simulink model "controllo_cascata_2019"  (R2019b)
settings: Solver=VariableStepAuto  StartTime=0.0  StopTime=5  RelTol=1e-3
values from neighbouring files (symbols this model uses):
  den = den{1}    [Km_con_filtri.m]    (also in fft_signal_analysis.m)
  Gden = Gden{1}    [controllore_mag_lin.m]
  Gnum = Gnum{1}    [controllore_mag_lin.m]
  ki = 2117.9265    [controller_el.m]    (also in controller_el_windup.m; controllore_el2.m = 104; controllore_mag_lin.m; validation_controller_freq.m = 2118)
  kp = 46.0161    [controller_el.m]    (also in controller_el_windup.m; controllore_el2.m = 0.15; controllore_mag_lin.m; validation_controller_freq.m = 46)
  Lc = 0.3935    [Model_Parameter.m]    (also in Model_Parameter_version2.m = 0.3708; Stima_dei_parametri_Rc_Lc.m = mean(Lc_vect))
  num = num{1}    [Km_con_filtri.m]    (also in fft_signal_analysis.m)
  Rtot = 9.089    [Model_Parameter.m]    (also in Model_Parameter_version2.m = 9.7585)
undefined symbols (not defined in the file or in its folder): den_ext, den_unico, dist, Gdclose, Gnclose, num_ext, num_unico, u0, x10, x1_eq
libraries: simulink x5
settings Model: Creator=lollo  LastModifiedBy=lollo
settings DebuggingCC: UnconnectedInputMsg=none  UnconnectedOutputMsg=none  UnconnectedLineMsg=none
settings ModelReferenceCC: EnableRefExpFcnMdlSchedulingChecks=off
settings RTWCC: Description=Generic Real-Time Target

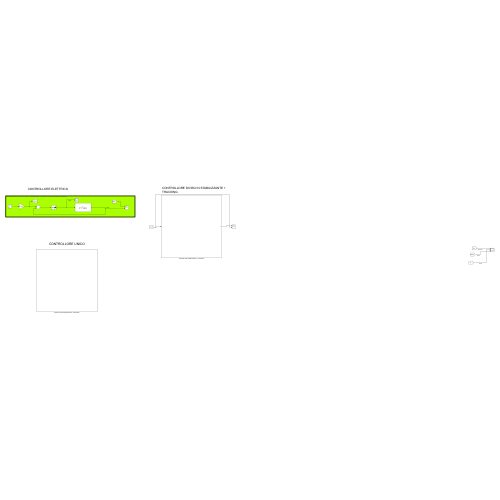
[thumbnail: Simulink's stored preview of the top-level diagram]
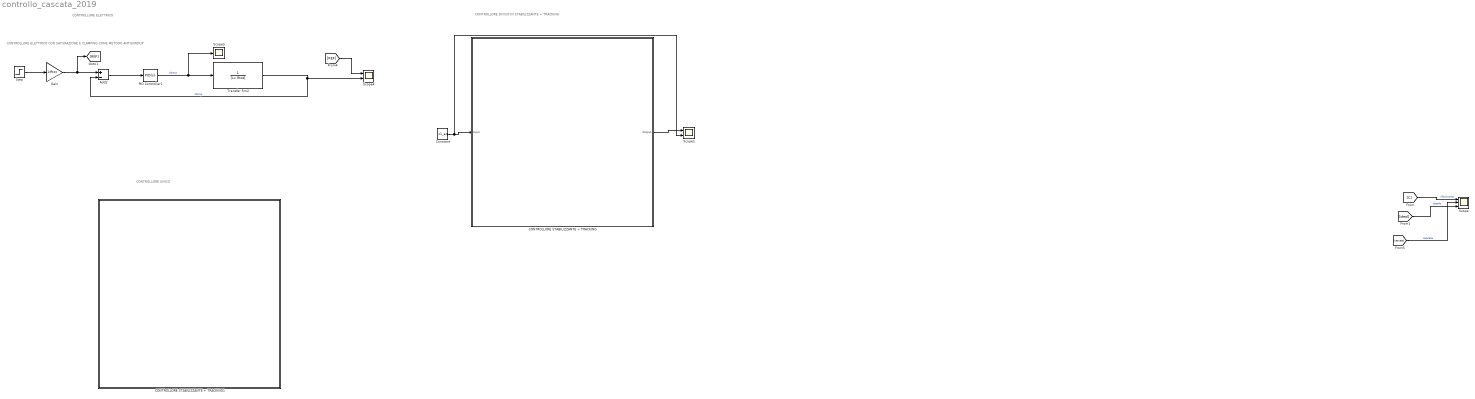
== system controllo_cascata_2019 ==
  note: CONTROLLORE UNICO
  note: CONTROLLORE ELETTRICO
  note: CONTROLLORE DIVISO IN STABILIZZANTE + TRACKING
  note: CONTROLLORE ELETTRICO CON SATURAZIONE E CLAMPING COME METODO ANTIWINDUP
  Add2 : Sum  Inputs=+-
  CONTROLLORE STABILIZZANTE + TRACKING : Subsystem
  CONTROLLORE STABILIZZANTE + TRACKING1 : Subsystem
  Constant : Constant  Value=x1_eq
  Gain : Gain  Gain=1/Rtot
  PID Controller1 : simulink/Continuous/PID Controller  Controller=PID  Form=Parallel  TimeDomain=Continuous-time  SampleTime=-1  IntegratorMethod=Forward Euler  FilterMethod=Forward Euler  ControllerParametersSource=internal  P=kp  I=ki  D=0  N=100  UseFilter=on  TunerSelectOption=Transfer Function Based (PID Tuner App)  InitialConditionSource=internal  InitialConditionForIntegrator=0  InitialConditionForFilter=0  DifferentiatorICPrevScaledInput=0  ExternalReset=none  TrackingMode=off  Kt=1  LimitOutput=on  UpperSaturationLimit=23  LowerSaturationLimit=-23  LinearizeAsGain=on  AntiWindupMode=clamping  Kb=1  POutMin=[]  POutMax=[]  IOutMin=[]  IOutMax=[]  DOutMin=[]  DOutMax=[]  NOutMin=[]  NOutMax=[]  SumOutMin=[]  SumOutMax=[]  SaturationOutMin=[]  SaturationOutMax=[]  PParamMin=[]  PParamMax=[]  IParamMin=[]  IParamMax=[]  DParamMin=[]  DParamMax=[]  NParamMin=[]  NParamMax=[]  KbParamMin=[]  KbParamMax=[]  KtParamMin=[]  KtParamMax=[]  KbOutMin=[]  KbOutMax=[]  KtOutMin=[]  KtOutMax=[]  IntegratorOutMin=[]  IntegratorOutMax=[]  FilterOutMin=[]  FilterOutMax=[]  SumI1OutMin=[]  SumI1OutMax=[]  SumI2OutMin=[]  SumI2OutMax=[]  SumI3OutMin=[]  SumI3OutMax=[]  SumI4OutMin=[]  SumI4OutMax=[]  SumDOutMin=[]  SumDOutMax=[]  DifferentiatorOutMin=[]  DifferentiatorOutMax=[]  FilterDiffOutCoefMin=[]  FilterDiffOutCoefMax=[]  ReciprocalOutMin=[]  ReciprocalOutMax=[]  SumDenOutMin=[]  SumDenOutMax=[]  SumNumOutMin=[]  SumNumOutMax=[]  DivideOutMin=[]  DivideOutMax=[]  IntegratorContinuousStateAttributes=''  IntegratorStateMustResolveToSignalObject=off  IntegratorRTWStateStorageClass=Auto  FilterContinuousStateAttributes=''  FilterStateMustResolveToSignalObject=off  FilterRTWStateStorageClass=Auto  ParallelPVariant=InternalParameters  IdealPVariant=Disabled  IVariant=InternalParameters  DVariant=InternalParameters  IntegratorVariant=Continuous  SatVariant=Enabled  AWVariant=ContClampingParallel  PCopyVariant=Disabled  TRVariant=Disabled  FdbkBlocksVariant=Forward  IdealPFdbkVariant=Disabled  SatFdbkVariant=Disabled  DerivativeFilterVariant=ContFilter  NVariant=InternalParameters  NCopyVariant=Disabled  FilterICVariant=InternalICsFilter  IntegratorICVariant=InternalICs  ExternalResetVariant=Disabled  TRSumVariant=Passthrough  SumFdbkVariant=Disabled  SumVariant=Sum_PID
  Scope : Scope  NumInputPorts=3
  Scope1 : Scope  NumInputPorts=2
  Scope4 : Scope  NumInputPorts=2
  Scope5 : Scope
  Step : Step  Time=0  After=10  SampleTime=0
  Transfer Fcn2 : TransferFcn  Denominator=[Lc Rtot]
  wires:
  Add2/1 -> PID Controller1/1
  PID Controller1/1 -> Scope5/1, Transfer Fcn2/1  "clamp"
  Transfer Fcn2/1 -> Scope4/2, Add2/2  "clamp"
  Step/1 -> Gain/1
  [REF] -> Scope4/1
  [C] -> Scope/1  "riferimenti"
  [ideal] -> Scope/3  "ideale"
  [cascata] -> Scope/2  "cascata"
  Gain/1 -> [REF], Add2/1
  Constant/1 -> Scope1/2, CONTROLLORE STABILIZZANTE + TRACKING/1(Input)
  CONTROLLORE STABILIZZANTE + TRACKING/1(Output) -> Scope1/1

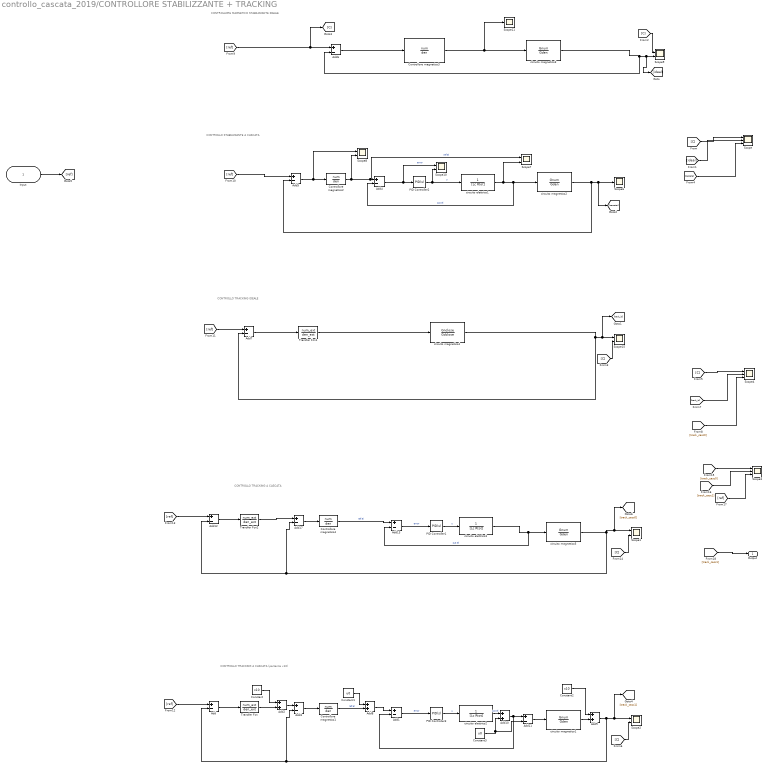
== system controllo_cascata_2019/CONTROLLORE STABILIZZANTE + TRACKING ==
  note: CONTROLLO STABILIZZANTE A CASCATA
  note: CONTROLLORE MAGNETICO STABILIZZANTE IDEALE
  note: CONTROLLO TRACKING A CASCATA (partenza x10)
  note: CONTROLLO TRACKING IDEALE
  note: CONTROLLO TRACKING A CASCATA
  Input : Inport
  Add{,1,3..7,11..13,17} (11 alike) : Sum  Inputs=+-
  Add{2,8..10} (4 alike) : Sum
  Constant : Constant  Value=x10
  Constant1 : Constant  Value=u0
  Constant2 : Constant  Value=x10
  Constant3 : Constant  Value=u0
  Controllore magnetico{1..4} (4 alike) : TransferFcn  Numerator=num  Denominator=den
  PID Controller1 : simulink/Continuous/PID Controller  Controller=PID  Form=Parallel  TimeDomain=Continuous-time  SampleTime=-1  IntegratorMethod=Forward Euler  FilterMethod=Forward Euler  ControllerParametersSource=internal  P=kp  I=ki  D=0  N=100  UseFilter=on  TunerSelectOption=Transfer Function Based (PID Tuner App)  InitialConditionSource=internal  InitialConditionForIntegrator=0  InitialConditionForFilter=0  DifferentiatorICPrevScaledInput=0  ExternalReset=none  TrackingMode=off  Kt=1  LimitOutput=on  UpperSaturationLimit=23  LowerSaturationLimit=-23  LinearizeAsGain=on  AntiWindupMode=clamping  Kb=1  POutMin=[]  POutMax=[]  IOutMin=[]  IOutMax=[]  DOutMin=[]  DOutMax=[]  NOutMin=[]  NOutMax=[]  SumOutMin=[]  SumOutMax=[]  SaturationOutMin=[]  SaturationOutMax=[]  PParamMin=[]  PParamMax=[]  IParamMin=[]  IParamMax=[]  DParamMin=[]  DParamMax=[]  NParamMin=[]  NParamMax=[]  KbParamMin=[]  KbParamMax=[]  KtParamMin=[]  KtParamMax=[]  KbOutMin=[]  KbOutMax=[]  KtOutMin=[]  KtOutMax=[]  IntegratorOutMin=[]  IntegratorOutMax=[]  FilterOutMin=[]  FilterOutMax=[]  SumI1OutMin=[]  SumI1OutMax=[]  SumI2OutMin=[]  SumI2OutMax=[]  SumI3OutMin=[]  SumI3OutMax=[]  SumI4OutMin=[]  SumI4OutMax=[]  SumDOutMin=[]  SumDOutMax=[]  DifferentiatorOutMin=[]  DifferentiatorOutMax=[]  FilterDiffOutCoefMin=[]  FilterDiffOutCoefMax=[]  ReciprocalOutMin=[]  ReciprocalOutMax=[]  SumDenOutMin=[]  SumDenOutMax=[]  SumNumOutMin=[]  SumNumOutMax=[]  DivideOutMin=[]  DivideOutMax=[]  IntegratorContinuousStateAttributes=''  IntegratorStateMustResolveToSignalObject=off  IntegratorRTWStateStorageClass=Auto  FilterContinuousStateAttributes=''  FilterStateMustResolveToSignalObject=off  FilterRTWStateStorageClass=Auto  ParallelPVariant=InternalParameters  IdealPVariant=Disabled  IVariant=InternalParameters  DVariant=InternalParameters  IntegratorVariant=Continuous  SatVariant=Enabled  AWVariant=ContClampingParallel  PCopyVariant=Disabled  TRVariant=Disabled  FdbkBlocksVariant=Forward  IdealPFdbkVariant=Disabled  SatFdbkVariant=Disabled  DerivativeFilterVariant=ContFilter  NVariant=InternalParameters  NCopyVariant=Disabled  FilterICVariant=InternalICsFilter  IntegratorICVariant=InternalICs  ExternalResetVariant=Disabled  TRSumVariant=Passthrough  SumFdbkVariant=Disabled  SumVariant=Sum_PID
  PID Controller2 : simulink/Continuous/PID Controller  Controller=PID  Form=Parallel  TimeDomain=Continuous-time  SampleTime=-1  IntegratorMethod=Forward Euler  FilterMethod=Forward Euler  ControllerParametersSource=internal  P=kp  I=ki  D=0  N=100  UseFilter=on  TunerSelectOption=Transfer Function Based (PID Tuner App)  InitialConditionSource=internal  InitialConditionForIntegrator=0  InitialConditionForFilter=0  DifferentiatorICPrevScaledInput=0  ExternalReset=none  TrackingMode=off  Kt=1  LimitOutput=on  UpperSaturationLimit=23  LowerSaturationLimit=-23  LinearizeAsGain=on  AntiWindupMode=clamping  Kb=1  POutMin=[]  POutMax=[]  IOutMin=[]  IOutMax=[]  DOutMin=[]  DOutMax=[]  NOutMin=[]  NOutMax=[]  SumOutMin=[]  SumOutMax=[]  SaturationOutMin=[]  SaturationOutMax=[]  PParamMin=[]  PParamMax=[]  IParamMin=[]  IParamMax=[]  DParamMin=[]  DParamMax=[]  NParamMin=[]  NParamMax=[]  KbParamMin=[]  KbParamMax=[]  KtParamMin=[]  KtParamMax=[]  KbOutMin=[]  KbOutMax=[]  KtOutMin=[]  KtOutMax=[]  IntegratorOutMin=[]  IntegratorOutMax=[]  FilterOutMin=[]  FilterOutMax=[]  SumI1OutMin=[]  SumI1OutMax=[]  SumI2OutMin=[]  SumI2OutMax=[]  SumI3OutMin=[]  SumI3OutMax=[]  SumI4OutMin=[]  SumI4OutMax=[]  SumDOutMin=[]  SumDOutMax=[]  DifferentiatorOutMin=[]  DifferentiatorOutMax=[]  FilterDiffOutCoefMin=[]  FilterDiffOutCoefMax=[]  ReciprocalOutMin=[]  ReciprocalOutMax=[]  SumDenOutMin=[]  SumDenOutMax=[]  SumNumOutMin=[]  SumNumOutMax=[]  DivideOutMin=[]  DivideOutMax=[]  IntegratorContinuousStateAttributes=''  IntegratorStateMustResolveToSignalObject=off  IntegratorRTWStateStorageClass=Auto  FilterContinuousStateAttributes=''  FilterStateMustResolveToSignalObject=off  FilterRTWStateStorageClass=Auto  ParallelPVariant=InternalParameters  IdealPVariant=Disabled  IVariant=InternalParameters  DVariant=InternalParameters  IntegratorVariant=Continuous  SatVariant=Enabled  AWVariant=ContClampingParallel  PCopyVariant=Disabled  TRVariant=Disabled  FdbkBlocksVariant=Forward  IdealPFdbkVariant=Disabled  SatFdbkVariant=Disabled  DerivativeFilterVariant=ContFilter  NVariant=InternalParameters  NCopyVariant=Disabled  FilterICVariant=InternalICsFilter  IntegratorICVariant=InternalICs  ExternalResetVariant=Disabled  TRSumVariant=Passthrough  SumFdbkVariant=Disabled  SumVariant=Sum_PID
  PID Controller3 : simulink/Continuous/PID Controller  Controller=PID  Form=Parallel  TimeDomain=Continuous-time  SampleTime=-1  IntegratorMethod=Forward Euler  FilterMethod=Forward Euler  ControllerParametersSource=internal  P=kp  I=ki  D=0  N=100  UseFilter=on  TunerSelectOption=Transfer Function Based (PID Tuner App)  InitialConditionSource=internal  InitialConditionForIntegrator=0  InitialConditionForFilter=0  DifferentiatorICPrevScaledInput=0  ExternalReset=none  TrackingMode=off  Kt=1  LimitOutput=on  UpperSaturationLimit=23  LowerSaturationLimit=-23  LinearizeAsGain=on  AntiWindupMode=clamping  Kb=1  POutMin=[]  POutMax=[]  IOutMin=[]  IOutMax=[]  DOutMin=[]  DOutMax=[]  NOutMin=[]  NOutMax=[]  SumOutMin=[]  SumOutMax=[]  SaturationOutMin=[]  SaturationOutMax=[]  PParamMin=[]  PParamMax=[]  IParamMin=[]  IParamMax=[]  DParamMin=[]  DParamMax=[]  NParamMin=[]  NParamMax=[]  KbParamMin=[]  KbParamMax=[]  KtParamMin=[]  KtParamMax=[]  KbOutMin=[]  KbOutMax=[]  KtOutMin=[]  KtOutMax=[]  IntegratorOutMin=[]  IntegratorOutMax=[]  FilterOutMin=[]  FilterOutMax=[]  SumI1OutMin=[]  SumI1OutMax=[]  SumI2OutMin=[]  SumI2OutMax=[]  SumI3OutMin=[]  SumI3OutMax=[]  SumI4OutMin=[]  SumI4OutMax=[]  SumDOutMin=[]  SumDOutMax=[]  DifferentiatorOutMin=[]  DifferentiatorOutMax=[]  FilterDiffOutCoefMin=[]  FilterDiffOutCoefMax=[]  ReciprocalOutMin=[]  ReciprocalOutMax=[]  SumDenOutMin=[]  SumDenOutMax=[]  SumNumOutMin=[]  SumNumOutMax=[]  DivideOutMin=[]  DivideOutMax=[]  IntegratorContinuousStateAttributes=''  IntegratorStateMustResolveToSignalObject=off  IntegratorRTWStateStorageClass=Auto  FilterContinuousStateAttributes=''  FilterStateMustResolveToSignalObject=off  FilterRTWStateStorageClass=Auto  ParallelPVariant=InternalParameters  IdealPVariant=Disabled  IVariant=InternalParameters  DVariant=InternalParameters  IntegratorVariant=Continuous  SatVariant=Enabled  AWVariant=ContClampingParallel  PCopyVariant=Disabled  TRVariant=Disabled  FdbkBlocksVariant=Forward  IdealPFdbkVariant=Disabled  SatFdbkVariant=Disabled  DerivativeFilterVariant=ContFilter  NVariant=InternalParameters  NCopyVariant=Disabled  FilterICVariant=InternalICsFilter  IntegratorICVariant=InternalICs  ExternalResetVariant=Disabled  TRSumVariant=Passthrough  SumFdbkVariant=Disabled  SumVariant=Sum_PID
  Scope : Scope  NumInputPorts=3
  Scope{1..2,7..10,15} (7 alike) : Scope  NumInputPorts=2
  Scope11 : Scope
  Scope3 : Scope  NumInputPorts=3
  Scope4 : Scope  NumInputPorts=3
  Scope6 : Scope
  Transfer Fcn : TransferFcn  Numerator=num_ext  Denominator=den_ext
  Transfer Fcn1 : TransferFcn  Numerator=num_ext  Denominator=den_ext
  Transfer Fcn2 : TransferFcn  Numerator=num_ext  Denominator=den_ext
  circuito elettrico1 : TransferFcn  Denominator=[Lc Rtot]
  circuito elettrico2 : TransferFcn  Denominator=[Lc Rtot]
  circuito elettrico3 : TransferFcn  Denominator=[Lc Rtot]
  circuito magnetico{1..3,5} (4 alike) : TransferFcn  Numerator=Gnum  Denominator=Gden
  circuito magnetico4 : TransferFcn  Numerator=Gnclose  Denominator=Gdclose
  Output : Outport
  wires:
  circuito magnetico2/1 -> Add5/2, [cascata], Scope6/1
  circuito elettrico1/1 -> Scope7/2, Add4/2, circuito magnetico2/1  "out el"
  Add4/1 -> Scope10/1, PID Controller2/1  "error"
  Controllore magnetico2/1 -> Scope8/2, Scope7/1, Add4/1  "ref el"
  PID Controller3/1 -> circuito elettrico2/1  "u"
  [ref] -> Add/1
  Add5/1 -> Scope8/1, Controllore magnetico2/1
  Transfer Fcn1/1 -> circuito magnetico4/1
  Add3/1 -> Controllore magnetico1/1
  Add/1 -> Transfer Fcn/1
  [ref] -> Add5/1
  circuito magnetico4/1 -> Add7/2, [track_id], Scope15/1
  PID Controller2/1 -> Scope10/2, circuito elettrico1/1  "u"
  Add6/1 -> Controllore magnetico3/1
  [ref] -> [C], Add6/1
  circuito magnetico3/1 -> Add6/2, [ideal], Scope9/2
  Controllore magnetico3/1 -> Scope11/1, circuito magnetico3/1
  Add1/1 -> PID Controller3/1  "error"
  [C] -> Scope9/1
  [ref] -> Add7/1
  [C] -> Scope15/2
  Add7/1 -> Transfer Fcn1/1
  [C] -> Scope2/2
  [C] -> Scope/1
  [ideal] -> Scope/2
  [cascata] -> Scope/3
  [C] -> Scope4/1
  [track_id] -> Scope4/2
  [track_casc0] -> Scope4/3
  Input/1 -> [ref]
  Transfer Fcn/1 -> Add2/2
  Add2/1 -> Add3/1
  Constant/1 -> Add2/1
  Add8/1 -> Add1/1
  Controllore magnetico1/1 -> Add8/2  "ref el"
  Constant1/1 -> Add8/1
  Add9/1 -> [track_casc1], Scope2/1, Add3/2, Add/2
  circuito magnetico1/1 -> Add9/2
  Constant2/1 -> Add9/1
  Add11/1 -> circuito magnetico1/1
  circuito elettrico2/1 -> Add10/1  "out el"
  Add10/1 -> Add1/2, Add11/1
  Constant3/1 -> Add11/2, Add10/2
  [ref] -> Add12/1
  Controllore magnetico4/1 -> Add13/1  "ref el"
  circuito elettrico3/1 -> Add13/2, circuito magnetico5/1  "out el"
  circuito magnetico5/1 -> [track_casc0], Scope1/1, Add17/2, Add12/2
  Transfer Fcn2/1 -> Add17/1
  Add12/1 -> Transfer Fcn2/1
  [C] -> Scope1/2
  Add17/1 -> Controllore magnetico4/1
  PID Controller1/1 -> circuito elettrico3/1  "u"
  Add13/1 -> PID Controller1/1  "error"
  [track_casc0] -> Scope3/1
  [track_casc1] -> Scope3/2
  [ref] -> Scope3/3
  [track_casc1] -> Output/1

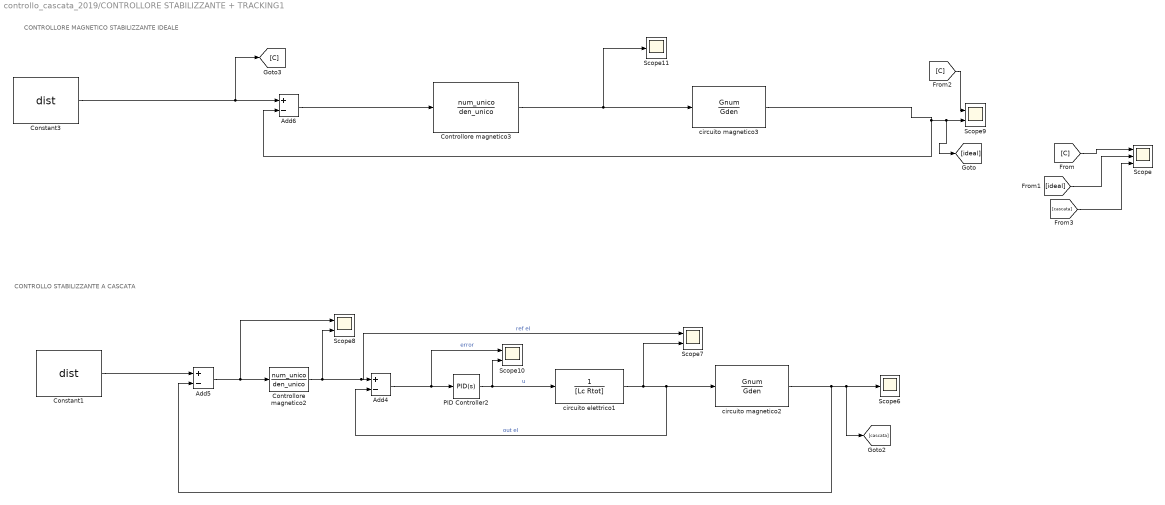
== system controllo_cascata_2019/CONTROLLORE STABILIZZANTE + TRACKING1 ==
  note: CONTROLLO STABILIZZANTE A CASCATA
  note: CONTROLLORE MAGNETICO STABILIZZANTE IDEALE
  Add4 : Sum  Inputs=+-
  Add5 : Sum  Inputs=+-
  Add6 : Sum  Inputs=+-
  Constant1 : Constant  Value=dist
  Constant3 : Constant  Value=dist
  Controllore magnetico2 : TransferFcn  Numerator=num_unico  Denominator=den_unico
  Controllore magnetico3 : TransferFcn  Numerator=num_unico  Denominator=den_unico
  PID Controller2 : simulink/Continuous/PID Controller  Controller=PID  Form=Parallel  TimeDomain=Continuous-time  SampleTime=-1  IntegratorMethod=Forward Euler  FilterMethod=Forward Euler  ControllerParametersSource=internal  P=kp  I=ki  D=0  N=100  UseFilter=on  TunerSelectOption=Transfer Function Based (PID Tuner App)  InitialConditionSource=internal  InitialConditionForIntegrator=0  InitialConditionForFilter=0  DifferentiatorICPrevScaledInput=0  ExternalReset=none  TrackingMode=off  Kt=1  LimitOutput=on  UpperSaturationLimit=23  LowerSaturationLimit=-23  LinearizeAsGain=on  AntiWindupMode=clamping  Kb=1  POutMin=[]  POutMax=[]  IOutMin=[]  IOutMax=[]  DOutMin=[]  DOutMax=[]  NOutMin=[]  NOutMax=[]  SumOutMin=[]  SumOutMax=[]  SaturationOutMin=[]  SaturationOutMax=[]  PParamMin=[]  PParamMax=[]  IParamMin=[]  IParamMax=[]  DParamMin=[]  DParamMax=[]  NParamMin=[]  NParamMax=[]  KbParamMin=[]  KbParamMax=[]  KtParamMin=[]  KtParamMax=[]  KbOutMin=[]  KbOutMax=[]  KtOutMin=[]  KtOutMax=[]  IntegratorOutMin=[]  IntegratorOutMax=[]  FilterOutMin=[]  FilterOutMax=[]  SumI1OutMin=[]  SumI1OutMax=[]  SumI2OutMin=[]  SumI2OutMax=[]  SumI3OutMin=[]  SumI3OutMax=[]  SumI4OutMin=[]  SumI4OutMax=[]  SumDOutMin=[]  SumDOutMax=[]  DifferentiatorOutMin=[]  DifferentiatorOutMax=[]  FilterDiffOutCoefMin=[]  FilterDiffOutCoefMax=[]  ReciprocalOutMin=[]  ReciprocalOutMax=[]  SumDenOutMin=[]  SumDenOutMax=[]  SumNumOutMin=[]  SumNumOutMax=[]  DivideOutMin=[]  DivideOutMax=[]  IntegratorContinuousStateAttributes=''  IntegratorStateMustResolveToSignalObject=off  IntegratorRTWStateStorageClass=Auto  FilterContinuousStateAttributes=''  FilterStateMustResolveToSignalObject=off  FilterRTWStateStorageClass=Auto  ParallelPVariant=InternalParameters  IdealPVariant=Disabled  IVariant=InternalParameters  DVariant=InternalParameters  IntegratorVariant=Continuous  SatVariant=Enabled  AWVariant=ContClampingParallel  PCopyVariant=Disabled  TRVariant=Disabled  FdbkBlocksVariant=Forward  IdealPFdbkVariant=Disabled  SatFdbkVariant=Disabled  DerivativeFilterVariant=ContFilter  NVariant=InternalParameters  NCopyVariant=Disabled  FilterICVariant=InternalICsFilter  IntegratorICVariant=InternalICs  ExternalResetVariant=Disabled  TRSumVariant=Passthrough  SumFdbkVariant=Disabled  SumVariant=Sum_PID
  Scope : Scope  NumInputPorts=3
  Scope{7..10} (4 alike) : Scope  NumInputPorts=2
  Scope11 : Scope
  Scope6 : Scope
  circuito elettrico1 : TransferFcn  Denominator=[Lc Rtot]
  circuito magnetico2 : TransferFcn  Numerator=Gnum  Denominator=Gden
  circuito magnetico3 : TransferFcn  Numerator=Gnum  Denominator=Gden
  wires:
  circuito magnetico2/1 -> Add5/2, [cascata], Scope6/1
  circuito elettrico1/1 -> Scope7/2, Add4/2, circuito magnetico2/1  "out el"
  Add4/1 -> Scope10/1, PID Controller2/1  "error"
  Controllore magnetico2/1 -> Scope8/2, Scope7/1, Add4/1  "ref el"
  Add5/1 -> Scope8/1, Controllore magnetico2/1
  Constant1/1 -> Add5/1
  PID Controller2/1 -> Scope10/2, circuito elettrico1/1  "u"
  Add6/1 -> Controllore magnetico3/1
  Constant3/1 -> [C], Add6/1
  circuito magnetico3/1 -> Add6/2, [ideal], Scope9/2
  Controllore magnetico3/1 -> Scope11/1, circuito magnetico3/1
  [C] -> Scope9/1
  ? -> ?
  [C] -> Scope/1
  [ideal] -> Scope/2
  [cascata] -> Scope/3
